simulink model "VehMot"  (R2018a)
settings: configuration reference "cs_ert" (kept outside this file)
settings Model: DataDictionary=VehMot.sldd  Creator=zhoutinglin  LastModifiedBy=zhoutinglin

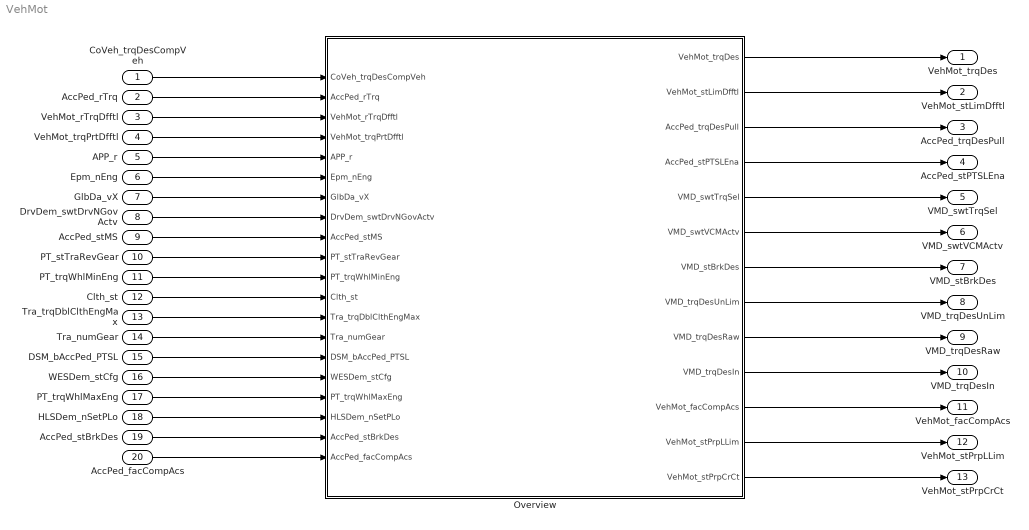
== system VehMot ==
  CoVeh_trqDesCompVeh : Inport
  AccPed_rTrq : Inport  Port=2
  VehMot_rTrqDfftl : Inport  Port=3
  VehMot_trqPrtDfftl : Inport  Port=4
  APP_r : Inport  Port=5
  Epm_nEng : Inport  Port=6
  GlbDa_vX : Inport  Port=7
  DrvDem_swtDrvNGovActv : Inport  Port=8
  AccPed_stMS : Inport  Port=9
  PT_stTraRevGear : Inport  Port=10
  PT_trqWhlMinEng : Inport  Port=11
  Clth_st : Inport  Port=12
  Tra_trqDblClthEngMax : Inport  Port=13
  Tra_numGear : Inport  Port=14
  DSM_bAccPed_PTSL : Inport  Port=15
  WESDem_stCfg : Inport  Port=16
  PT_trqWhlMaxEng : Inport  Port=17
  HLSDem_nSetPLo : Inport  Port=18
  AccPed_stBrkDes : Inport  Port=19
  AccPed_facCompAcs : Inport  Port=20
  Overview : Subsystem
  VehMot_trqDes : Outport
  VehMot_stLimDfftl : Outport  Port=2
  AccPed_trqDesPull : Outport  Port=3
  AccPed_stPTSLEna : Outport  Port=4
  VMD_swtTrqSel : Outport  Port=5
  VMD_swtVCMActv : Outport  Port=6
  VMD_stBrkDes : Outport  Port=7
  VMD_trqDesUnLim : Outport  Port=8
  VMD_trqDesRaw : Outport  Port=9
  VMD_trqDesIn : Outport  Port=10
  VehMot_facCompAcs : Outport  Port=11
  VehMot_stPrpLLim : Outport  Port=12
  VehMot_stPrpCrCt : Outport  Port=13
  wires:
  CoVeh_trqDesCompVeh/1 -> Overview/1(CoVeh_trqDesCompVeh)
  AccPed_rTrq/1 -> Overview/2(AccPed_rTrq)
  VehMot_rTrqDfftl/1 -> Overview/3(VehMot_rTrqDfftl)
  VehMot_trqPrtDfftl/1 -> Overview/4(VehMot_trqPrtDfftl)
  APP_r/1 -> Overview/5(APP_r)
  Epm_nEng/1 -> Overview/6(Epm_nEng)
  GlbDa_vX/1 -> Overview/7(GlbDa_vX)
  DrvDem_swtDrvNGovActv/1 -> Overview/8(DrvDem_swtDrvNGovActv)
  AccPed_stMS/1 -> Overview/9(AccPed_stMS)
  PT_stTraRevGear/1 -> Overview/10(PT_stTraRevGear)
  PT_trqWhlMinEng/1 -> Overview/11(PT_trqWhlMinEng)
  Clth_st/1 -> Overview/12(Clth_st)
  Tra_trqDblClthEngMax/1 -> Overview/13(Tra_trqDblClthEngMax)
  Tra_numGear/1 -> Overview/14(Tra_numGear)
  DSM_bAccPed_PTSL/1 -> Overview/15(DSM_bAccPed_PTSL)
  WESDem_stCfg/1 -> Overview/16(WESDem_stCfg)
  PT_trqWhlMaxEng/1 -> Overview/17(PT_trqWhlMaxEng)
  HLSDem_nSetPLo/1 -> Overview/18(HLSDem_nSetPLo)
  AccPed_stBrkDes/1 -> Overview/19(AccPed_stBrkDes)
  AccPed_facCompAcs/1 -> Overview/20(AccPed_facCompAcs)
  Overview/1(VehMot_trqDes) -> VehMot_trqDes/1
  Overview/2(VehMot_stLimDfftl) -> VehMot_stLimDfftl/1
  Overview/3(AccPed_trqDesPull) -> AccPed_trqDesPull/1
  Overview/4(AccPed_stPTSLEna) -> AccPed_stPTSLEna/1
  Overview/5(VMD_swtTrqSel) -> VMD_swtTrqSel/1
  Overview/6(VMD_swtVCMActv) -> VMD_swtVCMActv/1
  Overview/7(VMD_stBrkDes) -> VMD_stBrkDes/1
  Overview/8(VMD_trqDesUnLim) -> VMD_trqDesUnLim/1
  Overview/9(VMD_trqDesRaw) -> VMD_trqDesRaw/1
  Overview/10(VMD_trqDesIn) -> VMD_trqDesIn/1
  Overview/11(VehMot_facCompAcs) -> VehMot_facCompAcs/1
  Overview/12(VehMot_stPrpLLim) -> VehMot_stPrpLLim/1
  Overview/13(VehMot_stPrpCrCt) -> VehMot_stPrpCrCt/1

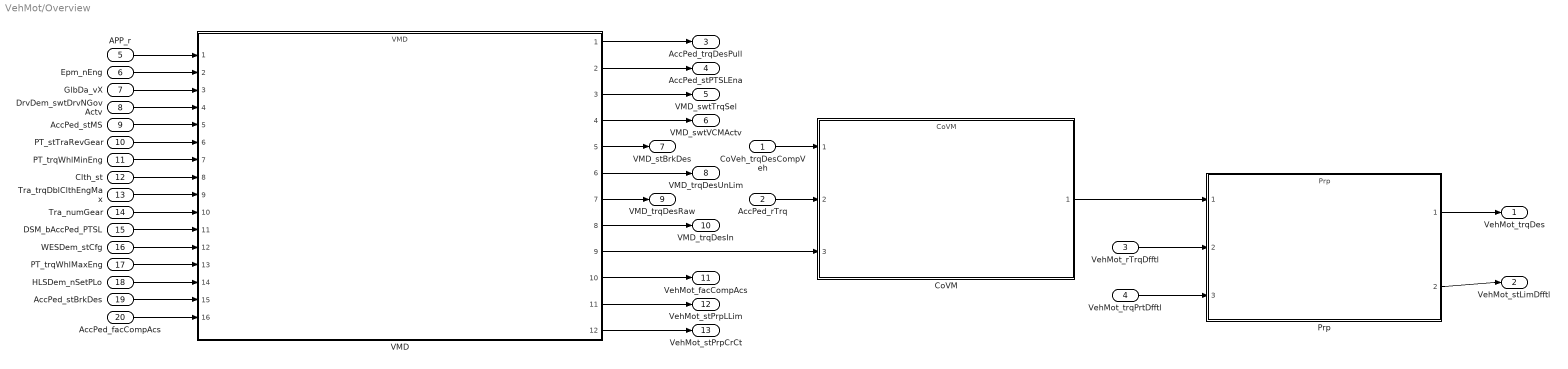
== system VehMot/Overview ==
  CoVeh_trqDesCompVeh : Inport
  AccPed_rTrq : Inport  Port=2
  VehMot_rTrqDfftl : Inport  Port=3
  VehMot_trqPrtDfftl : Inport  Port=4
  APP_r : Inport  Port=5
  Epm_nEng : Inport  Port=6
  GlbDa_vX : Inport  Port=7
  DrvDem_swtDrvNGovActv : Inport  Port=8
  AccPed_stMS : Inport  Port=9
  PT_stTraRevGear : Inport  Port=10
  PT_trqWhlMinEng : Inport  Port=11
  Clth_st : Inport  Port=12
  Tra_trqDblClthEngMax : Inport  Port=13
  Tra_numGear : Inport  Port=14
  DSM_bAccPed_PTSL : Inport  Port=15
  WESDem_stCfg : Inport  Port=16
  PT_trqWhlMaxEng : Inport  Port=17
  HLSDem_nSetPLo : Inport  Port=18
  AccPed_stBrkDes : Inport  Port=19
  AccPed_facCompAcs : Inport  Port=20
  CoVM : ModelReference  ModelNameDialog=CoVM  SimulationMode=Normal  ModelReferenceVersion=1.2
  Prp : ModelReference  ModelNameDialog=Prp  SimulationMode=Normal  ModelReferenceVersion=1.2
  VMD : ModelReference  ModelNameDialog=VMD  SimulationMode=Normal  ModelReferenceVersion=1.5
  VehMot_trqDes : Outport
  VehMot_stLimDfftl : Outport  Port=2
  AccPed_trqDesPull : Outport  Port=3
  AccPed_stPTSLEna : Outport  Port=4
  VMD_swtTrqSel : Outport  Port=5
  VMD_swtVCMActv : Outport  Port=6
  VMD_stBrkDes : Outport  Port=7
  VMD_trqDesUnLim : Outport  Port=8
  VMD_trqDesRaw : Outport  Port=9
  VMD_trqDesIn : Outport  Port=10
  VehMot_facCompAcs : Outport  Port=11
  VehMot_stPrpLLim : Outport  Port=12
  VehMot_stPrpCrCt : Outport  Port=13
  wires:
  VMD/9 -> CoVM/3
  CoVM/1 -> Prp/1
  CoVeh_trqDesCompVeh/1 -> CoVM/1
  AccPed_rTrq/1 -> CoVM/2
  VehMot_rTrqDfftl/1 -> Prp/2
  VehMot_trqPrtDfftl/1 -> Prp/3
  Prp/1 -> VehMot_trqDes/1
  Prp/2 -> VehMot_stLimDfftl/1
  APP_r/1 -> VMD/1
  Epm_nEng/1 -> VMD/2
  GlbDa_vX/1 -> VMD/3
  DrvDem_swtDrvNGovActv/1 -> VMD/4
  AccPed_stMS/1 -> VMD/5
  PT_stTraRevGear/1 -> VMD/6
  PT_trqWhlMinEng/1 -> VMD/7
  Clth_st/1 -> VMD/8
  Tra_trqDblClthEngMax/1 -> VMD/9
  Tra_numGear/1 -> VMD/10
  DSM_bAccPed_PTSL/1 -> VMD/11
  WESDem_stCfg/1 -> VMD/12
  PT_trqWhlMaxEng/1 -> VMD/13
  HLSDem_nSetPLo/1 -> VMD/14
  AccPed_stBrkDes/1 -> VMD/15
  AccPed_facCompAcs/1 -> VMD/16
  VMD/1 -> AccPed_trqDesPull/1
  VMD/2 -> AccPed_stPTSLEna/1
  VMD/3 -> VMD_swtTrqSel/1
  VMD/4 -> VMD_swtVCMActv/1
  VMD/5 -> VMD_stBrkDes/1
  VMD/6 -> VMD_trqDesUnLim/1
  VMD/7 -> VMD_trqDesRaw/1
  VMD/8 -> VMD_trqDesIn/1
  VMD/10 -> VehMot_facCompAcs/1
  VMD/11 -> VehMot_stPrpLLim/1
  VMD/12 -> VehMot_stPrpCrCt/1
